simulink model "QAM"  (R2016a)
settings: Solver=VariableStepAuto  StartTime=0.0  StopTime=1  RelTol=1e-3
libraries: commsrccod2 x6, dspsigops x4, simulink x3, dsparch4 x2, commchan3 x1, commsink2 x1, commseqgen3 x1
settings Model: Creator=hp  LastModifiedBy=hp

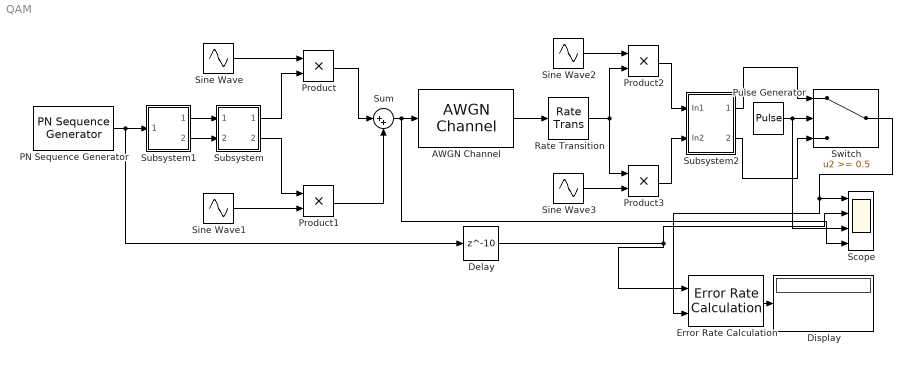
== system QAM ==
  AWGN Channel : commchan3/AWGN Channel  InputProcessing=Inherited (this choice will be removed - see release notes)  seed=67  noiseMode="Signal to noise ratio  (Eb/No)"  EbNodB=50  EsNodB=10  SNRdB=30  bitsPerSym=1  Ps=1  Tsym=1  variance=1
  Delay : Delay  DelayLength=10  InitialCondition=0
  Display : Display
  Error Rate Calculation : commsink2/Error Rate Calculation  N=8  st_delay=0  cp_mode=Entire frame  subframe=[]  PMode=Port  WsName=ErrorVec  RsMode2=off  stop=off  numErr=100  maxBits=1e6
  PN Sequence Generator : commseqgen3/PN Sequence Generator  poly=[1 0 0 0 0 1 1]  ini_sta=[0 0 0 0 0 1]  outBitMaskSource=Dialog parameter  shift=0  outVarSiz=off  maxOutSizeMode=Dialog parameter  maxOutSize=[10 1]  Ts=1/1000  sampPerFrame=1  reset=off  bitPackedOutputs=off  outDataType=double  numPackedBits=8  bitPackDataSigned=off  bitPackedOutDType=double
  Product{,1..3} (4 alike) : Product
  Pulse Generator : DiscretePulseGenerator  Period=10  PulseWidth=5  SampleTime=1/5000
  Rate Transition : RateTransition  OutPortSampleTimeOpt=Multiple of input port sample time  OutPortSampleTime=1/1000
  Scope : Scope  NumInputPorts=4
  Sine Wave : Sin  Frequency=5000*2*pi  Phase=pi/2  SampleTime=1/50000
  Sine Wave1 : Sin  Frequency=10000*pi  SampleTime=1/50000
  Sine Wave2 : Sin  Frequency=5000*2*pi  Phase=pi/2  SampleTime=1/50000
  Sine Wave3 : Sin  Frequency=5000*2*pi  SampleTime=1/50000
  Subsystem : Subsystem
  Subsystem1 : Subsystem
  Subsystem2 : Subsystem
  Sum : Sum  Inputs=|++  AccumDataTypeStr=double  OutDataTypeStr=double
  Switch : Switch  Threshold=0.5
  wires:
  Subsystem1/1(Out1) -> Subsystem/1(In1)
  Subsystem1/2(Out2) -> Subsystem/2(In2)
  Subsystem/1(Out1) -> Product/2
  Product/1 -> Sum/1
  Sine Wave/1 -> Product/1
  Sine Wave1/1 -> Product1/2
  Subsystem/2(Out2) -> Product1/1
  Product1/1 -> Sum/2
  Sum/1 -> Scope/4, AWGN Channel/1
  AWGN Channel/1 -> Rate Transition/1
  Sine Wave2/1 -> Product2/1
  Sine Wave3/1 -> Product3/2
  Product2/1 -> Subsystem2/1(In1)
  Product3/1 -> Subsystem2/2(In2)
  Pulse Generator/1 -> Scope/3, Switch/2
  Subsystem2/1(Out1) -> Switch/1
  Subsystem2/2(Out2) -> Switch/3
  Switch/1 -> Error Rate Calculation/2, Scope/1
  Error Rate Calculation/1 -> Display/1
  Rate Transition/1 -> Product3/1, Product2/2
  PN Sequence Generator/1 -> Delay/1, Subsystem1/1(In1)
  Delay/1 -> Error Rate Calculation/1, Scope/2

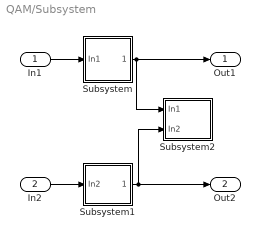
== system QAM/Subsystem ==
  In1 : Inport
  In2 : Inport  Port=2
  Subsystem : Subsystem
  Subsystem1 : Subsystem
  Subsystem2 : Subsystem
  Out1 : Outport
  Out2 : Outport  Port=2
  wires:
  In1/1 -> Subsystem/1(In1)
  In2/1 -> Subsystem1/1(In2)
  Subsystem/1(Out1) -> Subsystem2/1(In1), Out1/1
  Subsystem1/1(Out2) -> Subsystem2/2(In2), Out2/1

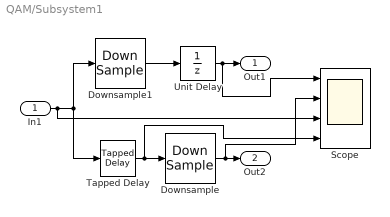
== system QAM/Subsystem1 ==
  In1 : Inport
  Downsample : DownSample
  Downsample1 : DownSample  RateOptions=Allow multirate processing
  Scope : Scope  NumInputPorts=4
  Tapped Delay : simulink/Discrete/Tapped Delay  vinit=0.0  samptime=1/1000  NumDelays=-1  DelayOrder=Oldest  includeCurrent=off
  Unit Delay : UnitDelay  SampleTime=1/500
  Out1 : Outport
  Out2 : Outport  Port=2
  wires:
  Downsample1/1 -> Unit Delay/1
  Tapped Delay/1 -> Scope/4, Downsample/1
  Downsample/1 -> Scope/2, Out2/1
  Unit Delay/1 -> Scope/1, Out1/1
  In1/1 -> Scope/3, Tapped Delay/1, Downsample1/1

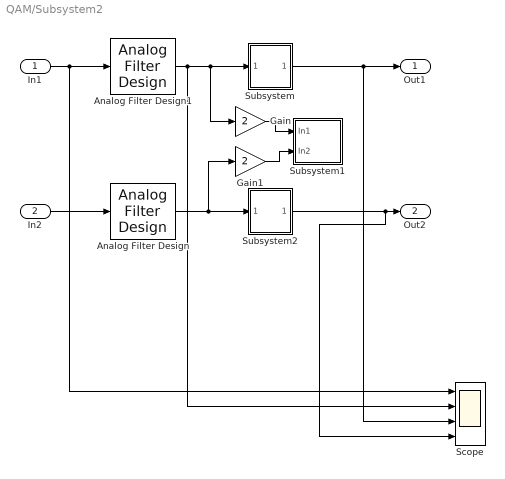
== system QAM/Subsystem2 ==
  In1 : Inport
  In2 : Inport  Port=2
  Analog Filter Design : dsparch4/Analog Filter Design  method=Bessel  filttype=Lowpass  N=8  Wlo=5000*pi  Whi=80  Rp=2  Rs=40
  Analog Filter Design1 : dsparch4/Analog Filter Design  method=Bessel  filttype=Lowpass  N=8  Wlo=5000*pi  Whi=80  Rp=2  Rs=40
  Gain : Gain  Gain=2
  Gain1 : Gain  Gain=2
  Scope : Scope  NumInputPorts=4
  Subsystem : Subsystem
  Subsystem1 : Subsystem
  Subsystem2 : Subsystem
  Out1 : Outport
  Out2 : Outport  Port=2
  wires:
  In1/1 -> Scope/1, Analog Filter Design1/1
  In2/1 -> Analog Filter Design/1
  Analog Filter Design/1 -> Subsystem2/1(In1), Gain1/1
  Analog Filter Design1/1 -> Scope/2, Gain/1, Subsystem/1(In1)
  Gain1/1 -> Subsystem1/2(In2)
  Gain/1 -> Subsystem1/1(In1)
  Subsystem/1(Out1) -> Scope/3, Out1/1
  Subsystem2/1(Out1) -> Scope/4, Out2/1

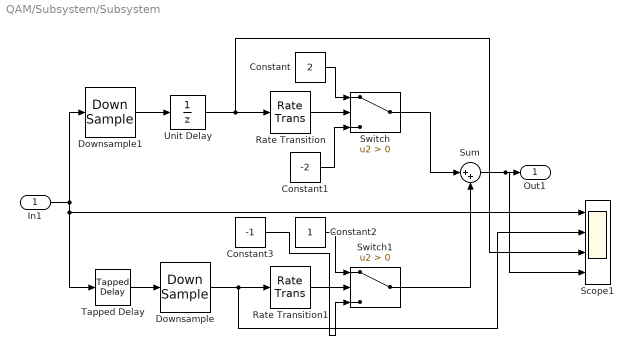
== system QAM/Subsystem/Subsystem ==
  In1 : Inport
  Constant : Constant  Value=2
  Constant1 : Constant  Value=-2
  Constant2 : Constant
  Constant3 : Constant  Value=-1
  Downsample : DownSample
  Downsample1 : DownSample
  Rate Transition : RateTransition  OutPortSampleTimeOpt=Multiple of input port sample time
  Rate Transition1 : RateTransition  OutPortSampleTimeOpt=Multiple of input port sample time
  Scope1 : Scope  NumInputPorts=4
  Sum : Sum  Inputs=|++
  Switch : Switch  Criteria=u2 > Threshold
  Switch1 : Switch  Criteria=u2 > Threshold
  Tapped Delay : simulink/Discrete/Tapped Delay  vinit=0.0  samptime=1/500  NumDelays=1  DelayOrder=Oldest  includeCurrent=off
  Unit Delay : UnitDelay  SampleTime=1/250
  Out1 : Outport
  wires:
  Downsample1/1 -> Unit Delay/1
  Tapped Delay/1 -> Downsample/1
  Unit Delay/1 -> Scope1/3, Rate Transition/1
  Constant/1 -> Switch/1
  Constant1/1 -> Switch/3
  Downsample/1 -> Scope1/2, Rate Transition1/1
  Constant2/1 -> Switch1/1
  Constant3/1 -> Switch1/3
  In1/1 -> Scope1/1, Tapped Delay/1, Downsample1/1
  Switch/1 -> Sum/1
  Switch1/1 -> Sum/2
  Sum/1 -> Scope1/4, Out1/1
  Rate Transition1/1 -> Switch1/2
  Rate Transition/1 -> Switch/2

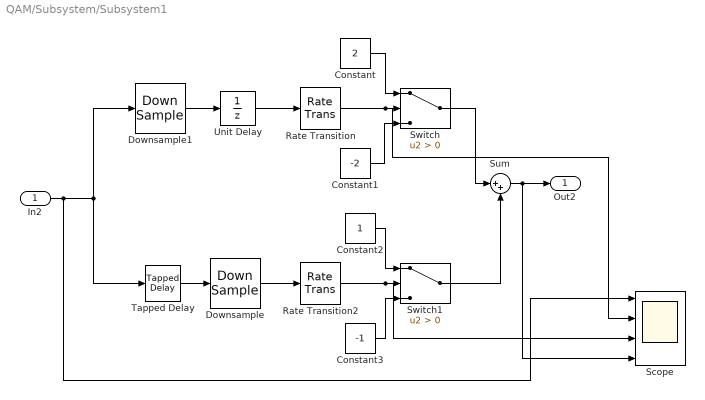
== system QAM/Subsystem/Subsystem1 ==
  In2 : Inport
  Constant : Constant  Value=2
  Constant1 : Constant  Value=-2
  Constant2 : Constant
  Constant3 : Constant  Value=-1
  Downsample : DownSample
  Downsample1 : DownSample
  Rate Transition : RateTransition  OutPortSampleTimeOpt=Multiple of input port sample time
  Rate Transition2 : RateTransition  OutPortSampleTimeOpt=Multiple of input port sample time
  Scope : Scope  NumInputPorts=4
  Sum : Sum  Inputs=|++
  Switch : Switch  Criteria=u2 > Threshold
  Switch1 : Switch  Criteria=u2 > Threshold
  Tapped Delay : simulink/Discrete/Tapped Delay  vinit=0.0  samptime=1/500  NumDelays=1  DelayOrder=Oldest  includeCurrent=off
  Unit Delay : UnitDelay  SampleTime=1/250
  Out2 : Outport
  wires:
  Downsample1/1 -> Unit Delay/1
  Tapped Delay/1 -> Downsample/1
  Unit Delay/1 -> Rate Transition/1
  Downsample/1 -> Rate Transition2/1
  Rate Transition/1 -> Scope/2, Switch/2
  Constant/1 -> Switch/1
  Constant1/1 -> Switch/3
  Rate Transition2/1 -> Scope/3, Switch1/2
  Constant2/1 -> Switch1/1
  Constant3/1 -> Switch1/3
  Sum/1 -> Scope/4, Out2/1
  Switch/1 -> Sum/1
  Switch1/1 -> Sum/2
  In2/1 -> Scope/1, Downsample1/1, Tapped Delay/1

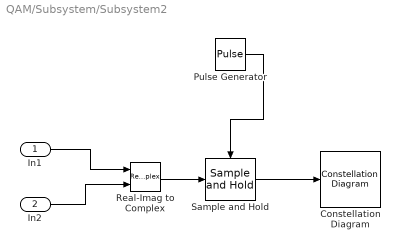
== system QAM/Subsystem/Subsystem2 ==
  In1 : Inport
  In2 : Inport  Port=2
  Constellation Diagram : ConstellationDiagram
  Pulse Generator : DiscretePulseGenerator  Period=10  PulseWidth=5  SampleTime=1/5000
  Real-Imag to Complex : RealImagToComplex
  Sample and Hold : dspsigops/Sample and Hold  trig=Rising edge  initCond=0  latchinput=off
  wires:
  In1/1 -> Real-Imag to Complex/1
  In2/1 -> Real-Imag to Complex/2
  Real-Imag to Complex/1 -> Sample and Hold/1
  Pulse Generator/1 -> Sample and Hold/Trigger
  Sample and Hold/1 -> Constellation Diagram/1

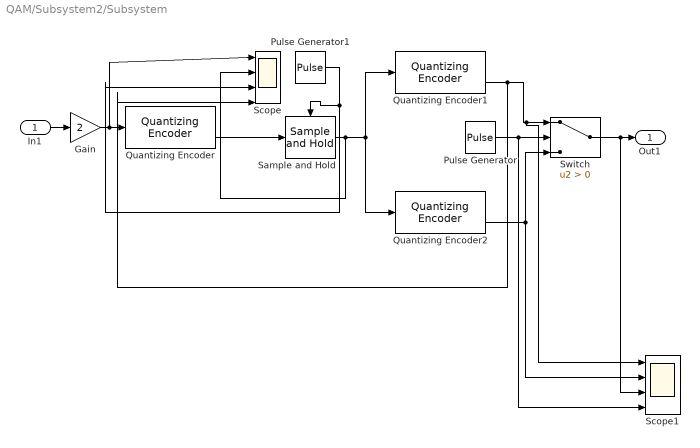
== system QAM/Subsystem2/Subsystem ==
  In1 : Inport
  Gain : Gain  Gain=2
  Pulse Generator : DiscretePulseGenerator  Period=10  PulseWidth=5  SampleTime=1/2500
  Pulse Generator1 : DiscretePulseGenerator  Period=10  PulseWidth=5  SampleTime=1/2500
  Quantizing Encoder : commsrccod2/Quantizing Encoder  partition=[-2.0 0 2.0]  codebook=[-3 -1 1 3]  idxDType=double
  Quantizing Encoder1 : commsrccod2/Quantizing Encoder  partition=[-2.0 0 2.0]  codebook=[0 0 1 1]  idxDType=double
  Quantizing Encoder2 : commsrccod2/Quantizing Encoder  partition=[-2.0 0 2.0]  codebook=[0 1 0 1]  idxDType=double
  Sample and Hold : dspsigops/Sample and Hold  trig=Rising edge  initCond=0  latchinput=off
  Scope : Scope  NumInputPorts=4
  Scope1 : Scope  NumInputPorts=4
  Switch : Switch  Criteria=u2 > Threshold  OutDataTypeStr=double
  Out1 : Outport
  wires:
  In1/1 -> Gain/1
  Gain/1 -> Scope/1, Quantizing Encoder/1
  Quantizing Encoder/2 -> Sample and Hold/1
  Sample and Hold/1 -> Scope/2, Quantizing Encoder2/1, Quantizing Encoder1/1
  Pulse Generator/1 -> Scope1/4, Switch/2
  Quantizing Encoder1/2 -> Scope/4, Scope1/1, Switch/1
  Quantizing Encoder2/2 -> Scope1/2, Switch/3
  Switch/1 -> Scope1/3, Out1/1
  Pulse Generator1/1 -> Scope/3, Sample and Hold/Trigger

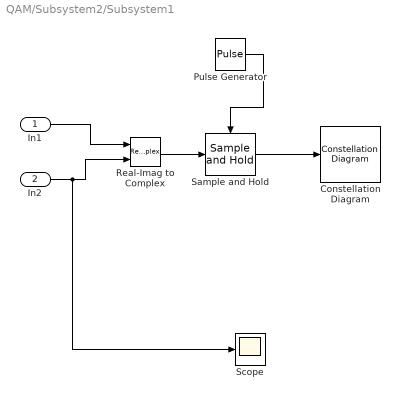
== system QAM/Subsystem2/Subsystem1 ==
  In1 : Inport
  In2 : Inport  Port=2
  Constellation Diagram : ConstellationDiagram
  Pulse Generator : DiscretePulseGenerator  Period=10  PulseWidth=5  SampleTime=1/5000
  Real-Imag to Complex : RealImagToComplex
  Sample and Hold : dspsigops/Sample and Hold  trig=Rising edge  initCond=0  latchinput=off
  Scope : Scope
  wires:
  In1/1 -> Real-Imag to Complex/1
  Real-Imag to Complex/1 -> Sample and Hold/1
  Pulse Generator/1 -> Sample and Hold/Trigger
  Sample and Hold/1 -> Constellation Diagram/1
  In2/1 -> Scope/1, Real-Imag to Complex/2

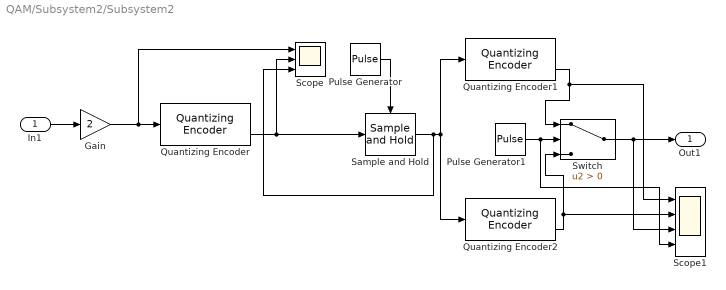
== system QAM/Subsystem2/Subsystem2 ==
  In1 : Inport
  Gain : Gain  Gain=2
  Pulse Generator : DiscretePulseGenerator  Period=10  PulseWidth=5  SampleTime=1/2500
  Pulse Generator1 : DiscretePulseGenerator  Period=10  PulseWidth=5  SampleTime=1/2500
  Quantizing Encoder : commsrccod2/Quantizing Encoder  partition=[-2.0 0 2.0]  codebook=[-3 -1 1 3]  idxDType=double
  Quantizing Encoder1 : commsrccod2/Quantizing Encoder  partition=[-2.0 0 2.0]  codebook=[0 0 1 1]  idxDType=double
  Quantizing Encoder2 : commsrccod2/Quantizing Encoder  partition=[-2.0 0 2.0]  codebook=[0 1 0 1]  idxDType=double
  Sample and Hold : dspsigops/Sample and Hold  trig=Rising edge  initCond=0  latchinput=off
  Scope : Scope  NumInputPorts=3
  Scope1 : Scope  NumInputPorts=4
  Switch : Switch  Criteria=u2 > Threshold
  Out1 : Outport
  wires:
  In1/1 -> Gain/1
  Gain/1 -> Scope/1, Quantizing Encoder/1
  Quantizing Encoder/2 -> Scope/2, Sample and Hold/1
  Pulse Generator/1 -> Sample and Hold/Trigger
  Pulse Generator1/1 -> Scope1/4, Switch/2
  Switch/1 -> Scope1/3, Out1/1
  Quantizing Encoder2/2 -> Switch/3, Scope1/2
  Sample and Hold/1 -> Scope/3, Quantizing Encoder1/1, Quantizing Encoder2/1
  Quantizing Encoder1/2 -> Scope1/1, Switch/1
